simulink model "Formation_FMS2"  (R2022b)
settings: Solver=FixedStepDiscrete  StartTime=0.0  StopTime=10.0  FixedStep=FMS_CONST.dt  RelTol=1e-3
values from neighbouring files (symbols this model uses):
  FMS_PARAM = Simulink.Parameter(FMS_PARAM_VALUE)    [fms_model_init.m]
  FORMATION_PARAM = Simulink.Parameter(FORMATION_PARAM_VALUE)    [fms_model_init.m]
undefined symbols (not defined in the file or in its folder): ax_cmd, ay_cmd, CONTROL_PARAM, DiscIntNeverNeededParam, PilotMode, state, VehicleState, vh_cmd
libraries: FC_Lib x51, simulink x16
(part 2 of 3)

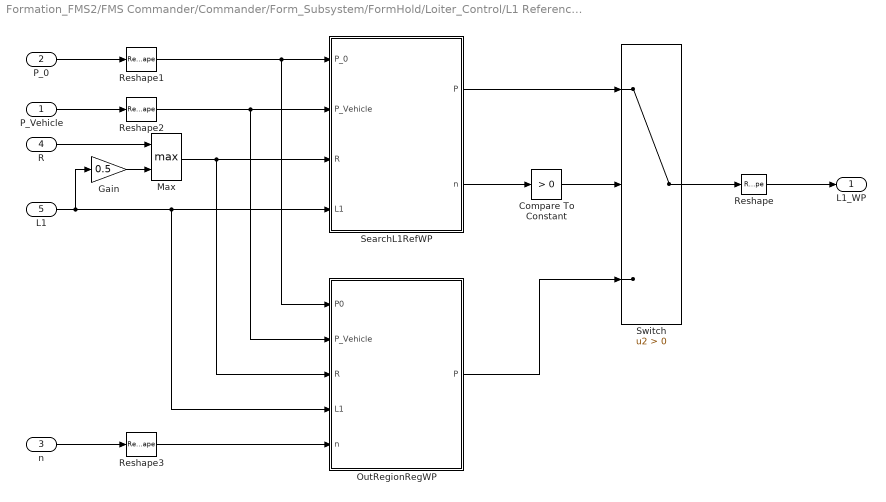
== system Formation_FMS2/FMS Commander/Commander/Form_Subsystem/FormHold/Loiter_Control/L1 Reference WP ==
  P_Vehicle : Inport
  P_0 : Inport  Port=2
  n : Inport  Port=3
  R : Inport  Port=4
  L1 : Inport  Port=5
  Compare To Constant : simulink/Logic and Bit Operations/Compare To Constant  relop=>  const=0  OutDataTypeStr=boolean
  Gain : Gain  Gain=0.5
  Max : MinMax  Function=max  Inputs=2
  OutRegionRegWP : MATLAB Function  TreatAsAtomicUnit=on
  Reshape : Reshape  OutputDimensionality=Customize  OutputDimensions=[2,1]
  Reshape1 : Reshape  OutputDimensionality=Column vector (2-D)
  Reshape2 : Reshape  OutputDimensionality=Column vector (2-D)
  Reshape3 : Reshape  OutputDimensionality=Column vector (2-D)
  SearchL1RefWP : MATLAB Function  TreatAsAtomicUnit=on
  Switch : Switch  Criteria=u2 > Threshold  SaturateOnIntegerOverflow=off  InputSameDT=off
  L1_WP : Outport  VectorParamsAs1DForOutWhenUnconnected=off
  wires:
  Reshape/1 -> L1_WP/1
  Compare To Constant/1 -> Switch/2
  SearchL1RefWP/2(n) -> Compare To Constant/1
  OutRegionRegWP/1(P) -> Switch/3
  Switch/1 -> Reshape/1
  SearchL1RefWP/1(P) -> Switch/1
  P_0/1 -> Reshape1/1
  P_Vehicle/1 -> Reshape2/1
  Max/1 -> OutRegionRegWP/3(R), SearchL1RefWP/3(R)
  L1/1 -> Gain/1, OutRegionRegWP/4(L1), SearchL1RefWP/4(L1)
  Reshape1/1 -> OutRegionRegWP/1(P0), SearchL1RefWP/1(P_0)
  Reshape2/1 -> OutRegionRegWP/2(P_Vehicle), SearchL1RefWP/2(P_Vehicle)
  n/1 -> Reshape3/1
  Reshape3/1 -> OutRegionRegWP/5(n)
  R/1 -> Max/1
  Gain/1 -> Max/2

== system Formation_FMS2/FMS Commander/Commander/Form_Subsystem/FormHold/Loiter_Control/L1_Core ==
  p_vehicle : Inport
  L1_WP : Inport  Port=2
  L1 : Inport  Port=3
  Vg : Inport  Port=4
  L1_Lateral_Acceleration : Subsystem
  Subtract : Sum  Inputs=+-
  ay_cmd_mPs2 : Outport  VectorParamsAs1DForOutWhenUnconnected=off
  wires:
  L1_WP/1 -> Subtract/1
  p_vehicle/1 -> Subtract/2
  L1/1 -> L1_Lateral_Acceleration/1(L1)
  Vg/1 -> L1_Lateral_Acceleration/2(Vg)
  Subtract/1 -> L1_Lateral_Acceleration/3(l1_path)
  L1_Lateral_Acceleration/1(l1_a_cmd) -> ay_cmd_mPs2/1

== system Formation_FMS2/FMS Commander/Commander/Form_Subsystem/FormHold/Loiter_Control/Reference_Point ==
  FMS_In : Inport
  Bus Selector1 : BusSelector  OutputSignals=Cmd_In.cur_waypoint
  Bus Selector2 : BusSelector  OutputSignals=INS_Out.vn,INS_Out.ve
  Bus Selector3 : BusSelector  OutputSignals=INS_Out.x_R,INS_Out.y_R
  Mux1 : Mux  Inputs=2
  Mux2 : Mux  Inputs=2
  Selector : Selector  InputPortWidth=3  IndexOptions=Index vector (dialog)  Indices=[1 2]  OutputSizes=1
  Vector Normalize : FC_Lib/Math/Vector Normalize
      settings: SourceProductName=Flight Control Toolbox
  start_vel : Delay  DelayLength=1  InitialConditionSource=Input port
      settings: InputPortMap=u0,p4
  p_vehicle : Outport  VectorParamsAs1DForOutWhenUnconnected=off
  p_0 : Outport  Port=2  VectorParamsAs1DForOutWhenUnconnected=off
  n : Outport  Port=3  VectorParamsAs1DForOutWhenUnconnected=off
  wires:
  Bus Selector2/2 -> Mux1/2  "<ve>"
  start_vel/1 -> Vector Normalize/1, start_vel/1
  Bus Selector2/1 -> Mux1/1  "<vn>"
  Vector Normalize/1 -> n/1
  FMS_In/1 -> Bus Selector3/1, Bus Selector2/1, Bus Selector1/1
  Mux1/1 -> start_vel/2
  Bus Selector3/1 -> Mux2/1  "<x_R>"
  Bus Selector3/2 -> Mux2/2  "<y_R>"
  Mux2/1 -> p_vehicle/1
  Bus Selector1/1 -> Selector/1  "<cur_waypoint>"
  Selector/1 -> p_0/1

== system Formation_FMS2/FMS Commander/Commander/Form_Subsystem/FormMission/FormMission_SubSystem/Formation_Controller ==
  note: TODO
  FMS_In : Inport
  Bus Selector : BusSelector  OutputSignals=Cmd_In.form_valid
  Bus Selector1 : BusSelector  OutputSignals=Formation_Cross.x_R,Formation_Cross.y_R,Formation_Cross.h_R,Formation_Cross.vn,Formation_Cross.ve,Formation_Cross.vd
  Bus Selector2 : BusSelector  OutputSignals=INS_Out.vn,INS_Out.ve
  Bus Selector3 : BusSelector  OutputSignals=INS_Out.psi
  Consensus Controller : FC_Lib/Fromation/Consensus Controller  uav_id=uav_id  adj_matrix=FORMATION_PARAM.ADJ_MARTIX  rel_x=FORMATION_PARAM.REL_X_MATRIX  rel_y=FORMATION_PARAM.REL_Y_MATRIX  rel_z=FORMATION_PARAM.REL_Z_MATRIX  damp=FORMATION_PARAM.LATERAL_DAMP  period=FORMATION_PARAM.LATERAL_PERIOD  vtrim=CONTROL_PARAM.FW_AIRSPD_TRIM  vmax=CONTROL_PARAM.FW_AIRSPD_MAX  vmin=CONTROL_PARAM.FW_AIRSPD_MIN  pos_kp=FORMATION_PARAM.FORM_POS_KP  vel_kp=FORMATION_PARAM.FORM_VEL_KP  pos_kd=FORMATION_PARAM.FORM_POS_KD
      settings: LibrarySourceBlock=|
      | simulink/User-Defined
      | Functions/MATLAB Function
  Mux : Mux  Inputs=2
  Saturation : Saturate  UpperLimit=inf  LowerLimit=-inf
  Saturation1 : Saturate  UpperLimit=inf  LowerLimit=-inf
  Saturation2 : Saturate  UpperLimit=inf  LowerLimit=-inf
  Vector Concatenate : Concatenate  NumInputs=3  Mode=Multidimensional array  ConcatenateDimension=2
  Vector Concatenate1 : Concatenate  NumInputs=3  Mode=Multidimensional array  ConcatenateDimension=2
  ux_cmd : Outport
  uy_cmd : Outport  Port=2
  uz_cmd : Outport  Port=3
  wires:
  Bus Selector1/2 -> Vector Concatenate/2  "<y_R>"
  Bus Selector/1 -> Consensus Controller/1  "<form_valid>"
  Bus Selector1/4 -> Vector Concatenate1/1  "<vn>"
  Consensus Controller/3 -> Saturation2/1
  Bus Selector1/3 -> Vector Concatenate/3  "<h_R>"
  Vector Concatenate/1 -> Consensus Controller/2  "xyz_O_nx3"
  Bus Selector1/5 -> Vector Concatenate1/2  "<ve>"
  Bus Selector1/1 -> Vector Concatenate/1  "<x_R>"
  Vector Concatenate1/1 -> Consensus Controller/3  "vNED_O_nx3"
  Consensus Controller/2 -> Saturation1/1
  Bus Selector1/6 -> Vector Concatenate1/3  "<vd>"
  FMS_In/1 -> Bus Selector/1, Bus Selector1/1, Bus Selector3/1, Bus Selector2/1
  Consensus Controller/1 -> Saturation/1
  Saturation/1 -> ux_cmd/1
  Saturation1/1 -> uy_cmd/1
  Saturation2/1 -> uz_cmd/1
  Bus Selector2/1 -> Mux/1  "<vn>"
  Bus Selector2/2 -> Mux/2  "<ve>"
  Mux/1 -> Consensus Controller/4
  Bus Selector3/1 -> Consensus Controller/5  "<psi>"

== system Formation_FMS2/FMS Commander/Commander/Form_Subsystem/FormMission/FormMission_SubSystem/Leader_Controller ==
  FMS_In : Inport
  Airspeed Hold : Subsystem
  Altitude_Hold : Subsystem
  FormRadiusLimit : Subsystem
  Position Command : Subsystem
  ax_cmd : Outport
  ay_cmd : Outport  Port=2
  vh_cmd : Outport  Port=3
  wires:
  FMS_In/1 -> Airspeed Hold/1(FMS_In), Altitude_Hold/1(FMS_In), Position Command/1(FMS_In)
  Altitude_Hold/1(vh_cmd) -> vh_cmd/1
  Airspeed Hold/1(ax_cmd) -> ax_cmd/1
  Position Command/1(ay_cmd) -> FormRadiusLimit/1(u)
  FormRadiusLimit/1(y) -> ay_cmd/1

== system Formation_FMS2/FMS Commander/Commander/Hold/Loiter_Control/L1_Core/L1_Lateral_Acceleration ==
  L1 : Inport
  Vg : Inport  Port=2
  l1_path : Inport  Port=3
  Divide : Product  Inputs=*/
  Gain : Gain  Gain=2
  Included Angle : Subsystem
  Multiply1 : Product
  Saturation : Saturate  UpperLimit=pi/2  LowerLimit=-pi/2
  Sin : Trigonometry
  Square : Math  Operator=square  SignedPower=on
  Vector Modulus : FC_Lib/Math/Vector Modulus
      settings: SourceProductName=Flight Control Toolbox
  Vector Normalize : FC_Lib/Math/Vector Normalize
      settings: SourceProductName=Flight Control Toolbox
  Vector Normalize1 : FC_Lib/Math/Vector Normalize
      settings: SourceProductName=Flight Control Toolbox
  l1_a_cmd : Outport  VectorParamsAs1DForOutWhenUnconnected=off
  wires:
  Vector Normalize/1 -> Included Angle/1(vec1)
  Included Angle/1(angle_rad) -> Saturation/1  "L1_alpha"
  Multiply1/1 -> Divide/1
  Divide/1 -> l1_a_cmd/1  "l1_a_cmd"
  Vector Normalize1/1 -> Included Angle/2(vec2)
  Sin/1 -> Multiply1/1  "sin_alpha"
  l1_path/1 -> Vector Normalize1/1
  Saturation/1 -> Sin/1
  Vg/1 -> Vector Normalize/1, Vector Modulus/1
  Square/1 -> Gain/1
  Gain/1 -> Multiply1/2
  L1/1 -> Divide/2
  Vector Modulus/1 -> Square/1

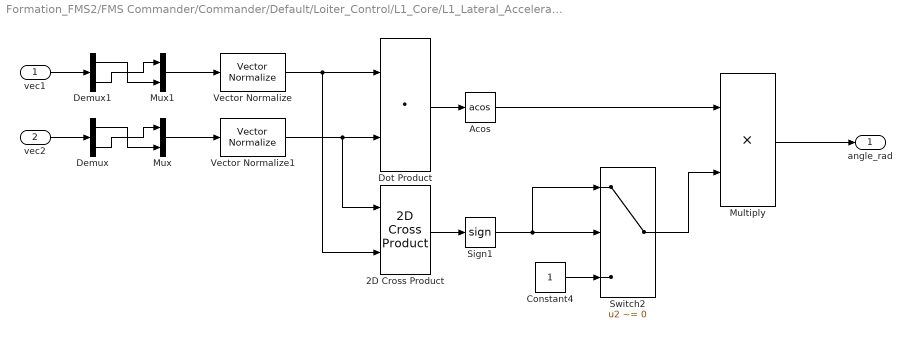
== system Formation_FMS2/FMS Commander/Commander/Default/Loiter_Control/L1_Core/L1_Lateral_Acceleration/Included Angle ==
  vec1 : Inport
  vec2 : Inport  Port=2
  2D Cross Product : FC_Lib/Math/2D Cross Product
      settings: SourceProductName=Flight Control Toolbox
  Acos : Trigonometry  Operator=acos
  Constant4 : Constant  OutDataTypeStr=single
  Demux : Demux  Outputs=2
  Demux1 : Demux  Outputs=2
  Dot Product : DotProduct  OutDataTypeStr=Inherit: Inherit via internal rule
  Multiply : Product
  Mux : Mux  Inputs=2
  Mux1 : Mux  Inputs=2
  Sign1 : Signum
  Switch2 : Switch  Criteria=u2 ~= 0  SaturateOnIntegerOverflow=off  InputSameDT=off
  Vector Normalize : FC_Lib/Math/Vector Normalize
      settings: SourceProductName=Flight Control Toolbox
  Vector Normalize1 : FC_Lib/Math/Vector Normalize
      settings: SourceProductName=Flight Control Toolbox
  angle_rad : Outport  VectorParamsAs1DForOutWhenUnconnected=off
  wires:
  Dot Product/1 -> Acos/1
  Demux1/1 -> Mux1/2
  Mux1/1 -> Vector Normalize/1
  Demux1/2 -> Mux1/1
  Sign1/1 -> Switch2/1, Switch2/2
  Vector Normalize1/1 -> Dot Product/2, 2D Cross Product/1
  Demux/2 -> Mux/1
  Vector Normalize/1 -> Dot Product/1, 2D Cross Product/2
  2D Cross Product/1 -> Sign1/1
  Multiply/1 -> angle_rad/1
  vec1/1 -> Demux1/1
  Demux/1 -> Mux/2
  Constant4/1 -> Switch2/3
  vec2/1 -> Demux/1
  Mux/1 -> Vector Normalize1/1
  Acos/1 -> Multiply/1
  Switch2/1 -> Multiply/2

== system Formation_FMS2/FMS Commander/Commander/Form_Subsystem/Default/Loiter_Control/L1_Core/L1_Lateral_Acceleration ==
  L1 : Inport
  Vg : Inport  Port=2
  l1_path : Inport  Port=3
  Divide : Product  Inputs=*/
  Gain : Gain  Gain=2
  Included Angle : Subsystem
  Multiply1 : Product
  Saturation : Saturate  UpperLimit=pi/2  LowerLimit=-pi/2
  Sin : Trigonometry
  Square : Math  Operator=square  SignedPower=on
  Vector Modulus : FC_Lib/Math/Vector Modulus
      settings: SourceProductName=Flight Control Toolbox
  Vector Normalize : FC_Lib/Math/Vector Normalize
      settings: SourceProductName=Flight Control Toolbox
  Vector Normalize1 : FC_Lib/Math/Vector Normalize
      settings: SourceProductName=Flight Control Toolbox
  l1_a_cmd : Outport  VectorParamsAs1DForOutWhenUnconnected=off
  wires:
  Vector Modulus/1 -> Square/1
  L1/1 -> Divide/2
  Gain/1 -> Multiply1/2
  Square/1 -> Gain/1
  Vg/1 -> Vector Modulus/1, Vector Normalize/1
  Saturation/1 -> Sin/1
  l1_path/1 -> Vector Normalize1/1
  Sin/1 -> Multiply1/1  "sin_alpha"
  Vector Normalize1/1 -> Included Angle/2(vec2)
  Divide/1 -> l1_a_cmd/1  "l1_a_cmd"
  Multiply1/1 -> Divide/1
  Included Angle/1(angle_rad) -> Saturation/1  "L1_alpha"
  Vector Normalize/1 -> Included Angle/1(vec1)

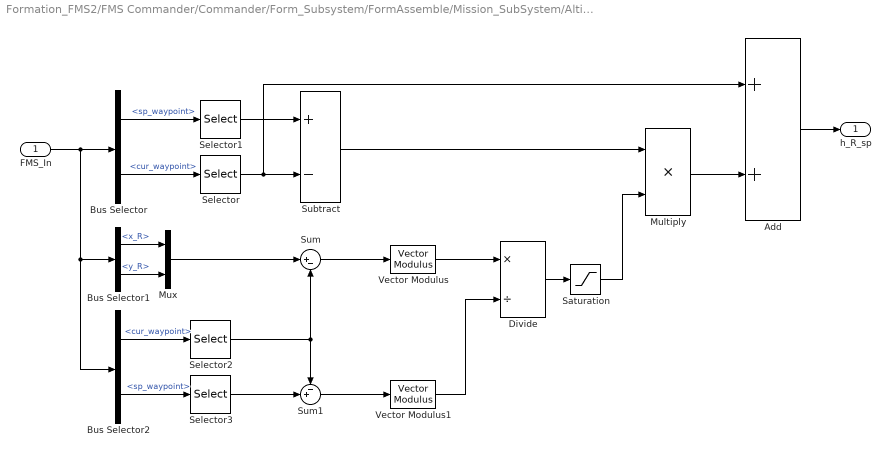
== system Formation_FMS2/FMS Commander/Commander/Form_Subsystem/FormAssemble/Mission_SubSystem/Altitude Control/Target Height ==
  FMS_In : Inport
  Add : Sum
  Bus Selector : BusSelector  OutputSignals=Cmd_In.sp_waypoint,Cmd_In.cur_waypoint
  Bus Selector1 : BusSelector  OutputSignals=INS_Out.x_R,INS_Out.y_R
  Bus Selector2 : BusSelector  OutputSignals=Cmd_In.cur_waypoint,Cmd_In.sp_waypoint
  Divide : Product  Inputs=*/
  Multiply : Product
  Mux : Mux  Inputs=2
  Saturation : Saturate  UpperLimit=1  LowerLimit=0
  Selector : Selector  InputPortWidth=3  IndexOptions=Index vector (dialog)  Indices=3  OutputSizes=1
  Selector1 : Selector  InputPortWidth=3  IndexOptions=Index vector (dialog)  Indices=3  OutputSizes=1
  Selector2 : Selector  InputPortWidth=3  IndexOptions=Index vector (dialog)  Indices=[1 2]  OutputSizes=1
  Selector3 : Selector  InputPortWidth=3  IndexOptions=Index vector (dialog)  Indices=[1 2]  OutputSizes=1
  Subtract : Sum  Inputs=+-
  Sum : Sum  Inputs=|+-
  Sum1 : Sum  Inputs=-+|
  Vector Modulus : FC_Lib/Math/Vector Modulus
      settings: SourceProductName=Flight Control Toolbox
  Vector Modulus1 : FC_Lib/Math/Vector Modulus
      settings: SourceProductName=Flight Control Toolbox
  h_R_sp : Outport  VectorParamsAs1DForOutWhenUnconnected=off
  wires:
  Multiply/1 -> Add/2
  Bus Selector1/1 -> Mux/1  "<x_R>"
  Bus Selector/1 -> Selector1/1  "<sp_waypoint>"
  Vector Modulus1/1 -> Divide/2
  Sum1/1 -> Vector Modulus1/1
  Sum/1 -> Vector Modulus/1
  Selector2/1 -> Sum1/1, Sum/2
  FMS_In/1 -> Bus Selector2/1, Bus Selector1/1, Bus Selector/1
  Bus Selector2/2 -> Selector3/1  "<sp_waypoint>"
  Vector Modulus/1 -> Divide/1
  Bus Selector1/2 -> Mux/2  "<y_R>"
  Bus Selector2/1 -> Selector2/1  "<cur_waypoint>"
  Selector1/1 -> Subtract/1
  Mux/1 -> Sum/1
  Subtract/1 -> Multiply/1
  Divide/1 -> Saturation/1
  Selector3/1 -> Sum1/2
  Bus Selector/2 -> Selector/1  "<cur_waypoint>"
  Selector/1 -> Add/1, Subtract/2
  Saturation/1 -> Multiply/2
  Add/1 -> h_R_sp/1

== system Formation_FMS2/FMS Commander/Commander/Form_Subsystem/FormAssemble/Mission_SubSystem/Position Command/L1 Control ==
  p1 : Inport
  p2 : Inport  Port=2
  p3 : Inport  Port=3
  FMS_In : Inport  Port=4
  Bus Selector1 : BusSelector  OutputSignals=INS_Out.vn,INS_Out.ve
  L1 : Constant  Value=FMS_PARAM.L1  OutDataTypeStr=single
  L1 Reference WP : Subsystem
  L1_Core : Subsystem
  Mux : Mux  Inputs=2
  Saturation1 : Saturate  UpperLimit=FMS_PARAM.ACC_Y_LIM  LowerLimit=-FMS_PARAM.ACC_Y_LIM
  ay_cmd_mPs2 : Outport  VectorParamsAs1DForOutWhenUnconnected=off
  wires:
  p3/1 -> L1_Core/1(p_vehicle), L1 Reference WP/3(P3)
  p2/1 -> L1 Reference WP/2(P2)
  p1/1 -> L1 Reference WP/1(P1)
  L1/1 -> L1_Core/3(L1), L1 Reference WP/4(L1)
  L1 Reference WP/1(L1_WP) -> L1_Core/2(L1_WP)  "L1_WP"
  Mux/1 -> L1_Core/4(Vg)
  Bus Selector1/1 -> Mux/1  "<vn>"
  Bus Selector1/2 -> Mux/2  "<ve>"
  FMS_In/1 -> Bus Selector1/1
  L1_Core/1(ay_cmd_mPs2) -> Saturation1/1
  Saturation1/1 -> ay_cmd_mPs2/1

== system Formation_FMS2/FMS Commander/Commander/Form_Subsystem/FormAssemble/Mission_SubSystem/Position Command/WayPoints ==
  note: P1: path start point
      | P2: path end point
      | P3: vehicle point
  FMS_In : Inport
  Bus Selector : BusSelector  OutputSignals=INS_Out.x_R,INS_Out.y_R
  Bus Selector1 : BusSelector  OutputSignals=Cmd_In.sp_waypoint
  Bus Selector2 : BusSelector  OutputSignals=Cmd_In.cur_waypoint
  Mux : Mux  Inputs=2
  Reshape : Reshape  OutputDimensionality=Customize  OutputDimensions=[2,1]
  Reshape1 : Reshape  OutputDimensionality=Customize  OutputDimensions=[2,1]
  Reshape2 : Reshape  OutputDimensionality=Customize  OutputDimensions=[2,1]
  Selector : Selector  InputPortWidth=3  IndexOptions=Index vector (dialog)  Indices=[1 2]  OutputSizes=1
  Selector1 : Selector  InputPortWidth=3  IndexOptions=Index vector (dialog)  Indices=[1 2]  OutputSizes=1
  p1 : Outport  VectorParamsAs1DForOutWhenUnconnected=off
  p2 : Outport  Port=2  VectorParamsAs1DForOutWhenUnconnected=off
  p3 : Outport  Port=3  VectorParamsAs1DForOutWhenUnconnected=off
  wires:
  Reshape2/1 -> p3/1
  Reshape1/1 -> p1/1
  Reshape/1 -> p2/1
  Bus Selector/2 -> Mux/2  "<y_R>"
  Bus Selector/1 -> Mux/1  "<x_R>"
  Mux/1 -> Reshape2/1
  FMS_In/1 -> Bus Selector2/1, Bus Selector1/1, Bus Selector/1
  Bus Selector1/1 -> Selector/1  "<sp_waypoint>"
  Selector/1 -> Reshape/1
  Bus Selector2/1 -> Selector1/1  "<cur_waypoint>"
  Selector1/1 -> Reshape1/1

== system Formation_FMS2/FMS Commander/Commander/Form_Subsystem/FormDisband/Loiter_Control/L1_Core/L1_Lateral_Acceleration ==
  L1 : Inport
  Vg : Inport  Port=2
  l1_path : Inport  Port=3
  Divide : Product  Inputs=*/
  Gain : Gain  Gain=2
  Included Angle : Subsystem
  Multiply1 : Product
  Saturation : Saturate  UpperLimit=pi/2  LowerLimit=-pi/2
  Sin : Trigonometry
  Square : Math  Operator=square  SignedPower=on
  Vector Modulus : FC_Lib/Math/Vector Modulus
      settings: SourceProductName=Flight Control Toolbox
  Vector Normalize : FC_Lib/Math/Vector Normalize
      settings: SourceProductName=Flight Control Toolbox
  Vector Normalize1 : FC_Lib/Math/Vector Normalize
      settings: SourceProductName=Flight Control Toolbox
  l1_a_cmd : Outport  VectorParamsAs1DForOutWhenUnconnected=off
  wires:
  Vector Modulus/1 -> Square/1
  L1/1 -> Divide/2
  Gain/1 -> Multiply1/2
  Square/1 -> Gain/1
  Vg/1 -> Vector Modulus/1, Vector Normalize/1
  Saturation/1 -> Sin/1
  l1_path/1 -> Vector Normalize1/1
  Sin/1 -> Multiply1/1  "sin_alpha"
  Vector Normalize1/1 -> Included Angle/2(vec2)
  Divide/1 -> l1_a_cmd/1  "l1_a_cmd"
  Multiply1/1 -> Divide/1
  Included Angle/1(angle_rad) -> Saturation/1  "L1_alpha"
  Vector Normalize/1 -> Included Angle/1(vec1)

== system Formation_FMS2/FMS Commander/Commander/Form_Subsystem/FormHold/Loiter_Control/L1_Core/L1_Lateral_Acceleration ==
  L1 : Inport
  Vg : Inport  Port=2
  l1_path : Inport  Port=3
  Divide : Product  Inputs=*/
  Gain : Gain  Gain=2
  Included Angle : Subsystem
  Multiply1 : Product
  Saturation : Saturate  UpperLimit=pi/2  LowerLimit=-pi/2
  Sin : Trigonometry
  Square : Math  Operator=square  SignedPower=on
  Vector Modulus : FC_Lib/Math/Vector Modulus
      settings: SourceProductName=Flight Control Toolbox
  Vector Normalize : FC_Lib/Math/Vector Normalize
      settings: SourceProductName=Flight Control Toolbox
  Vector Normalize1 : FC_Lib/Math/Vector Normalize
      settings: SourceProductName=Flight Control Toolbox
  l1_a_cmd : Outport  VectorParamsAs1DForOutWhenUnconnected=off
  wires:
  Vector Normalize/1 -> Included Angle/1(vec1)
  Included Angle/1(angle_rad) -> Saturation/1  "L1_alpha"
  Multiply1/1 -> Divide/1
  Divide/1 -> l1_a_cmd/1  "l1_a_cmd"
  Vector Normalize1/1 -> Included Angle/2(vec2)
  Sin/1 -> Multiply1/1  "sin_alpha"
  l1_path/1 -> Vector Normalize1/1
  Saturation/1 -> Sin/1
  Vg/1 -> Vector Normalize/1, Vector Modulus/1
  Square/1 -> Gain/1
  Gain/1 -> Multiply1/2
  L1/1 -> Divide/2
  Vector Modulus/1 -> Square/1

== system Formation_FMS2/FMS Commander/Commander/Form_Subsystem/FormMission/FormMission_SubSystem/Leader_Controller/Airspeed Hold ==
  FMS_In : Inport
  Bus Selector : BusSelector  OutputSignals=INS_Out.airspeed
  Constant : Constant  Value=FMS_PARAM.FW_AIRSPD_TRIM
  Gain : Gain  Gain=FMS_PARAM.AIRSPD_P
  Sum : Sum  Inputs=-+|
  ax_cmd : Outport
  wires:
  Sum/1 -> Gain/1  "v_error"
  Gain/1 -> ax_cmd/1  "ax_cmd"
  Constant/1 -> Sum/2
  FMS_In/1 -> Bus Selector/1
  Bus Selector/1 -> Sum/1  "<airspeed>"

== system Formation_FMS2/FMS Commander/Commander/Form_Subsystem/FormMission/FormMission_SubSystem/Leader_Controller/Altitude_Hold ==
  FMS_In : Inport
  Bus Selector2 : BusSelector  OutputSignals=INS_Out.h_R
  Constant : Constant  Value=FMS_PARAM.FW_HEIGHT_TRIM
  Delay : Delay  DelayLength=1  InitialConditionSource=Input port
      settings: InputPortMap=u0,p4
  Gain2 : Gain  Gain=FMS_PARAM.Z_P  OutDataTypeStr=single
  Saturation : Saturate  UpperLimit=CONTROL_PARAM.FW_T_CLMB_MAX  LowerLimit=-CONTROL_PARAM.FW_T_SINK_MAX
  Sum : Sum  Inputs=-+|
  vh_cmd : Outport  VectorParamsAs1DForOutWhenUnconnected=off
  wires:
  Gain2/1 -> Saturation/1
  Bus Selector2/1 -> Sum/1  "<h_R>"
  Sum/1 -> Gain2/1  "h_err_R"
  Delay/1 -> Sum/2, Delay/1  "h_cmd_R"
  FMS_In/1 -> Bus Selector2/1
  Saturation/1 -> vh_cmd/1
  Constant/1 -> Delay/2

== system Formation_FMS2/FMS Commander/Commander/Form_Subsystem/FormMission/FormMission_SubSystem/Leader_Controller/FormRadiusLimit ==
  note: R_{leader} > \frac{D_{lateral} \times V_{leader}}{min(V_{max} - V_{leader}, V_{leader} - V_{min})}
  u : Inport
  Divide : Product  Inputs=*/
  Gain : Gain  Gain=-1
  Satefy : Gain  Gain=FMS_PARAM.FW_RADIUS_RATIO
  Saturation Dynamic : simulink/Discontinuities/Saturation Dynamic  OutMin=[]  OutMax=[]  OutDataTypeStr=Inherit: Same as second input  OutDataType=fixdt(1, 16)  OutScaling=2^-10  DoSatur=off
  min_radius : MATLAB Function  TreatAsAtomicUnit=on  mask{dis_lat=FORMATION_PARAM.REL_Y_MATRIX, vtrim=CONTROL_PARAM.FW_AIRSPD_TRIM, vmax=CONTROL_PARAM.FW_AIRSPD_MAX, vmin=CONTROL_PARAM.FW_AIRSPD_MIN}
  v^2 : Constant  Value=CONTROL_PARAM.FW_AIRSPD_TRIM*CONTROL_PARAM.FW_AIRSPD_TRIM
  y : Outport
  wires:
  v^2/1 -> Divide/1
  Divide/1 -> Saturation Dynamic/1, Gain/1
  u/1 -> Saturation Dynamic/2
  Gain/1 -> Saturation Dynamic/3
  Saturation Dynamic/1 -> y/1
  Satefy/1 -> Divide/2
  min_radius/1(y) -> Satefy/1

== system Formation_FMS2/FMS Commander/Commander/Form_Subsystem/FormMission/FormMission_SubSystem/Leader_Controller/Position Command ==
  FMS_In : Inport
  L1 Control : Subsystem
  WayPoints : Subsystem
  ay_cmd : Outport  VectorParamsAs1DForOutWhenUnconnected=off
  wires:
  FMS_In/1 -> L1 Control/4(FMS_In), WayPoints/1(FMS_In)
  WayPoints/2(p2) -> L1 Control/2(p2)
  WayPoints/3(p3) -> L1 Control/3(p3)
  WayPoints/1(p1) -> L1 Control/1(p1)
  L1 Control/1(ay_cmd_mPs2) -> ay_cmd/1

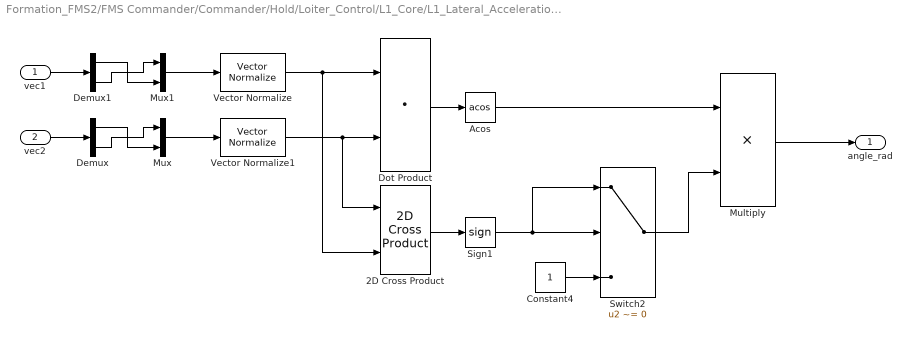
== system Formation_FMS2/FMS Commander/Commander/Hold/Loiter_Control/L1_Core/L1_Lateral_Acceleration/Included Angle ==
  vec1 : Inport
  vec2 : Inport  Port=2
  2D Cross Product : FC_Lib/Math/2D Cross Product
      settings: SourceProductName=Flight Control Toolbox
  Acos : Trigonometry  Operator=acos
  Constant4 : Constant  OutDataTypeStr=single
  Demux : Demux  Outputs=2
  Demux1 : Demux  Outputs=2
  Dot Product : DotProduct  OutDataTypeStr=Inherit: Inherit via internal rule
  Multiply : Product
  Mux : Mux  Inputs=2
  Mux1 : Mux  Inputs=2
  Sign1 : Signum
  Switch2 : Switch  Criteria=u2 ~= 0  SaturateOnIntegerOverflow=off  InputSameDT=off
  Vector Normalize : FC_Lib/Math/Vector Normalize
      settings: SourceProductName=Flight Control Toolbox
  Vector Normalize1 : FC_Lib/Math/Vector Normalize
      settings: SourceProductName=Flight Control Toolbox
  angle_rad : Outport  VectorParamsAs1DForOutWhenUnconnected=off
  wires:
  Switch2/1 -> Multiply/2
  Acos/1 -> Multiply/1
  Mux/1 -> Vector Normalize1/1
  vec2/1 -> Demux/1
  Constant4/1 -> Switch2/3
  Demux/1 -> Mux/2
  vec1/1 -> Demux1/1
  Multiply/1 -> angle_rad/1
  2D Cross Product/1 -> Sign1/1
  Vector Normalize/1 -> 2D Cross Product/2, Dot Product/1
  Demux/2 -> Mux/1
  Vector Normalize1/1 -> 2D Cross Product/1, Dot Product/2
  Sign1/1 -> Switch2/2, Switch2/1
  Demux1/2 -> Mux1/1
  Mux1/1 -> Vector Normalize/1
  Demux1/1 -> Mux1/2
  Dot Product/1 -> Acos/1

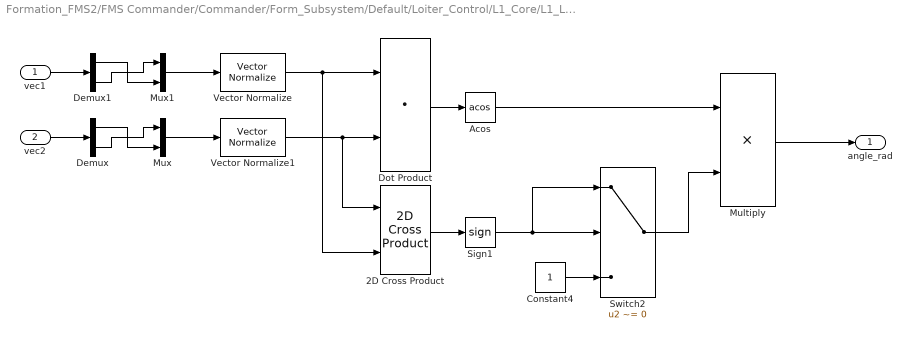
== system Formation_FMS2/FMS Commander/Commander/Form_Subsystem/Default/Loiter_Control/L1_Core/L1_Lateral_Acceleration/Included Angle ==
  vec1 : Inport
  vec2 : Inport  Port=2
  2D Cross Product : FC_Lib/Math/2D Cross Product
      settings: SourceProductName=Flight Control Toolbox
  Acos : Trigonometry  Operator=acos
  Constant4 : Constant  OutDataTypeStr=single
  Demux : Demux  Outputs=2
  Demux1 : Demux  Outputs=2
  Dot Product : DotProduct  OutDataTypeStr=Inherit: Inherit via internal rule
  Multiply : Product
  Mux : Mux  Inputs=2
  Mux1 : Mux  Inputs=2
  Sign1 : Signum
  Switch2 : Switch  Criteria=u2 ~= 0  SaturateOnIntegerOverflow=off  InputSameDT=off
  Vector Normalize : FC_Lib/Math/Vector Normalize
      settings: SourceProductName=Flight Control Toolbox
  Vector Normalize1 : FC_Lib/Math/Vector Normalize
      settings: SourceProductName=Flight Control Toolbox
  angle_rad : Outport  VectorParamsAs1DForOutWhenUnconnected=off
  wires:
  Dot Product/1 -> Acos/1
  Demux1/1 -> Mux1/2
  Mux1/1 -> Vector Normalize/1
  Demux1/2 -> Mux1/1
  Sign1/1 -> Switch2/1, Switch2/2
  Vector Normalize1/1 -> Dot Product/2, 2D Cross Product/1
  Demux/2 -> Mux/1
  Vector Normalize/1 -> Dot Product/1, 2D Cross Product/2
  2D Cross Product/1 -> Sign1/1
  Multiply/1 -> angle_rad/1
  vec1/1 -> Demux1/1
  Demux/1 -> Mux/2
  Constant4/1 -> Switch2/3
  vec2/1 -> Demux/1
  Mux/1 -> Vector Normalize1/1
  Acos/1 -> Multiply/1
  Switch2/1 -> Multiply/2

== system Formation_FMS2/FMS Commander/Commander/Form_Subsystem/FormAssemble/Mission_SubSystem/Position Command/L1 Control/L1 Reference WP ==
  P1 : Inport
  P2 : Inport  Port=2
  P3 : Inport  Port=3
  L1 : Inport  Port=4
  Compare To Constant : simulink/Logic and Bit Operations/Compare To Constant  relop=>=  const=0  OutDataTypeStr=boolean
  Compare To Constant1 : simulink/Logic and Bit Operations/Compare To Constant  relop=>  const=0  OutDataTypeStr=boolean
  NearbyRefWP : MATLAB Function  TreatAsAtomicUnit=on
  OutRegionRegWP : MATLAB Function  TreatAsAtomicUnit=on
  Reshape : Reshape  OutputDimensionality=Customize  OutputDimensions=[2,1]
  SearchL1RefWP : MATLAB Function  TreatAsAtomicUnit=on
  Switch : Switch  Criteria=u2 > Threshold  SaturateOnIntegerOverflow=off  InputSameDT=off
  Switch1 : Switch  Criteria=u2 > Threshold  SaturateOnIntegerOverflow=off  InputSameDT=off
  L1_WP : Outport  VectorParamsAs1DForOutWhenUnconnected=off
  wires:
  Reshape/1 -> L1_WP/1
  Compare To Constant/1 -> Switch/2
  NearbyRefWP/2(d) -> Compare To Constant1/1  "distance"
  SearchL1RefWP/2(u) -> Compare To Constant/1  "l1_u"
  Compare To Constant1/1 -> Switch1/2
  P1/1 -> SearchL1RefWP/1(P1), OutRegionRegWP/1(P1)
  P2/1 -> SearchL1RefWP/2(P2), NearbyRefWP/1(P2), OutRegionRegWP/2(P2)
  P3/1 -> NearbyRefWP/2(P3), SearchL1RefWP/3(P3), OutRegionRegWP/3(P3)
  Switch/1 -> Switch1/3
  L1/1 -> SearchL1RefWP/4(L1), NearbyRefWP/3(L1)
  OutRegionRegWP/1(P) -> Switch/3  "out_WP"
  Switch1/1 -> Reshape/1
  SearchL1RefWP/1(P) -> Switch/1  "L1_Ref_P"
  NearbyRefWP/1(P) -> Switch1/1  "NearbyWP"

== system Formation_FMS2/FMS Commander/Commander/Form_Subsystem/FormAssemble/Mission_SubSystem/Position Command/L1 Control/L1_Core ==
  p_vehicle : Inport
  L1_WP : Inport  Port=2
  L1 : Inport  Port=3
  Vg : Inport  Port=4
  L1_Lateral_Acceleration : Subsystem
  Subtract : Sum  Inputs=+-
  ay_cmd_mPs2 : Outport  VectorParamsAs1DForOutWhenUnconnected=off
  wires:
  L1_WP/1 -> Subtract/1
  p_vehicle/1 -> Subtract/2
  L1/1 -> L1_Lateral_Acceleration/1(L1)
  Vg/1 -> L1_Lateral_Acceleration/2(Vg)
  Subtract/1 -> L1_Lateral_Acceleration/3(l1_path)
  L1_Lateral_Acceleration/1(l1_a_cmd) -> ay_cmd_mPs2/1

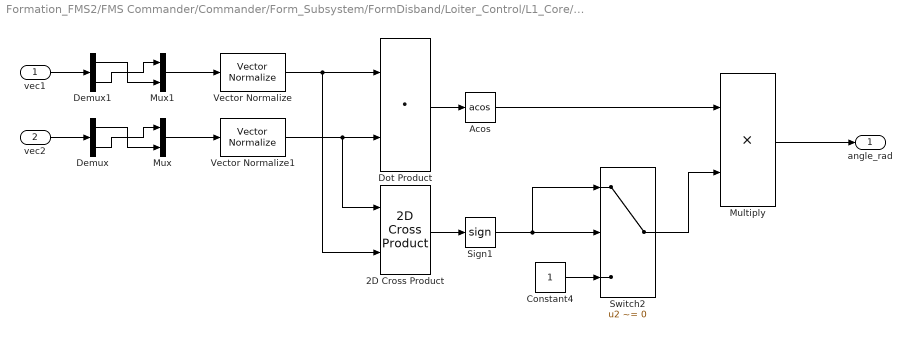
== system Formation_FMS2/FMS Commander/Commander/Form_Subsystem/FormDisband/Loiter_Control/L1_Core/L1_Lateral_Acceleration/Included Angle ==
  vec1 : Inport
  vec2 : Inport  Port=2
  2D Cross Product : FC_Lib/Math/2D Cross Product
      settings: SourceProductName=Flight Control Toolbox
  Acos : Trigonometry  Operator=acos
  Constant4 : Constant  OutDataTypeStr=single
  Demux : Demux  Outputs=2
  Demux1 : Demux  Outputs=2
  Dot Product : DotProduct  OutDataTypeStr=Inherit: Inherit via internal rule
  Multiply : Product
  Mux : Mux  Inputs=2
  Mux1 : Mux  Inputs=2
  Sign1 : Signum
  Switch2 : Switch  Criteria=u2 ~= 0  SaturateOnIntegerOverflow=off  InputSameDT=off
  Vector Normalize : FC_Lib/Math/Vector Normalize
      settings: SourceProductName=Flight Control Toolbox
  Vector Normalize1 : FC_Lib/Math/Vector Normalize
      settings: SourceProductName=Flight Control Toolbox
  angle_rad : Outport  VectorParamsAs1DForOutWhenUnconnected=off
  wires:
  Dot Product/1 -> Acos/1
  Demux1/1 -> Mux1/2
  Mux1/1 -> Vector Normalize/1
  Demux1/2 -> Mux1/1
  Sign1/1 -> Switch2/1, Switch2/2
  Vector Normalize1/1 -> Dot Product/2, 2D Cross Product/1
  Demux/2 -> Mux/1
  Vector Normalize/1 -> Dot Product/1, 2D Cross Product/2
  2D Cross Product/1 -> Sign1/1
  Multiply/1 -> angle_rad/1
  vec1/1 -> Demux1/1
  Demux/1 -> Mux/2
  Constant4/1 -> Switch2/3
  vec2/1 -> Demux/1
  Mux/1 -> Vector Normalize1/1
  Acos/1 -> Multiply/1
  Switch2/1 -> Multiply/2

== system Formation_FMS2/FMS Commander/Commander/Form_Subsystem/FormHold/Loiter_Control/L1_Core/L1_Lateral_Acceleration/Included Angle ==
  vec1 : Inport
  vec2 : Inport  Port=2
  2D Cross Product : FC_Lib/Math/2D Cross Product
      settings: SourceProductName=Flight Control Toolbox
  Acos : Trigonometry  Operator=acos
  Constant4 : Constant  OutDataTypeStr=single
  Demux : Demux  Outputs=2
  Demux1 : Demux  Outputs=2
  Dot Product : DotProduct  OutDataTypeStr=Inherit: Inherit via internal rule
  Multiply : Product
  Mux : Mux  Inputs=2
  Mux1 : Mux  Inputs=2
  Sign1 : Signum
  Switch2 : Switch  Criteria=u2 ~= 0  SaturateOnIntegerOverflow=off  InputSameDT=off
  Vector Normalize : FC_Lib/Math/Vector Normalize
      settings: SourceProductName=Flight Control Toolbox
  Vector Normalize1 : FC_Lib/Math/Vector Normalize
      settings: SourceProductName=Flight Control Toolbox
  angle_rad : Outport  VectorParamsAs1DForOutWhenUnconnected=off
  wires:
  Switch2/1 -> Multiply/2
  Acos/1 -> Multiply/1
  Mux/1 -> Vector Normalize1/1
  vec2/1 -> Demux/1
  Constant4/1 -> Switch2/3
  Demux/1 -> Mux/2
  vec1/1 -> Demux1/1
  Multiply/1 -> angle_rad/1
  2D Cross Product/1 -> Sign1/1
  Vector Normalize/1 -> 2D Cross Product/2, Dot Product/1
  Demux/2 -> Mux/1
  Vector Normalize1/1 -> 2D Cross Product/1, Dot Product/2
  Sign1/1 -> Switch2/2, Switch2/1
  Demux1/2 -> Mux1/1
  Mux1/1 -> Vector Normalize/1
  Demux1/1 -> Mux1/2
  Dot Product/1 -> Acos/1

== system Formation_FMS2/FMS Commander/Commander/Form_Subsystem/FormMission/FormMission_SubSystem/Leader_Controller/Position Command/L1 Control ==
  p1 : Inport
  p2 : Inport  Port=2
  p3 : Inport  Port=3
  FMS_In : Inport  Port=4
  Bus Selector1 : BusSelector  OutputSignals=INS_Out.vn,INS_Out.ve
  L1 : Constant  Value=FMS_PARAM.L1  OutDataTypeStr=single
  L1 Reference WP : Subsystem
  L1_Core : Subsystem
  Mux : Mux  Inputs=2
  Saturation1 : Saturate  UpperLimit=FMS_PARAM.ACC_Y_LIM  LowerLimit=-FMS_PARAM.ACC_Y_LIM
  ay_cmd_mPs2 : Outport  VectorParamsAs1DForOutWhenUnconnected=off
  wires:
  p3/1 -> L1_Core/1(p_vehicle), L1 Reference WP/3(P3)
  p2/1 -> L1 Reference WP/2(P2)
  p1/1 -> L1 Reference WP/1(P1)
  L1/1 -> L1_Core/3(L1), L1 Reference WP/4(L1)
  L1 Reference WP/1(L1_WP) -> L1_Core/2(L1_WP)  "L1_WP"
  Mux/1 -> L1_Core/4(Vg)
  Bus Selector1/1 -> Mux/1  "<vn>"
  Bus Selector1/2 -> Mux/2  "<ve>"
  FMS_In/1 -> Bus Selector1/1
  L1_Core/1(ay_cmd_mPs2) -> Saturation1/1
  Saturation1/1 -> ay_cmd_mPs2/1

== system Formation_FMS2/FMS Commander/Commander/Form_Subsystem/FormMission/FormMission_SubSystem/Leader_Controller/Position Command/WayPoints ==
  note: P1: path start point
      | P2: path end point
      | P3: vehicle point
  FMS_In : Inport
  Bus Selector : BusSelector  OutputSignals=INS_Out.x_R,INS_Out.y_R
  Bus Selector1 : BusSelector  OutputSignals=Cmd_In.sp_waypoint
  Bus Selector2 : BusSelector  OutputSignals=Cmd_In.cur_waypoint
  Mux : Mux  Inputs=2
  Reshape : Reshape  OutputDimensionality=Customize  OutputDimensions=[2,1]
  Reshape1 : Reshape  OutputDimensionality=Customize  OutputDimensions=[2,1]
  Reshape2 : Reshape  OutputDimensionality=Customize  OutputDimensions=[2,1]
  Selector : Selector  InputPortWidth=3  IndexOptions=Index vector (dialog)  Indices=[1 2]  OutputSizes=1
  Selector1 : Selector  InputPortWidth=3  IndexOptions=Index vector (dialog)  Indices=[1 2]  OutputSizes=1
  p1 : Outport  VectorParamsAs1DForOutWhenUnconnected=off
  p2 : Outport  Port=2  VectorParamsAs1DForOutWhenUnconnected=off
  p3 : Outport  Port=3  VectorParamsAs1DForOutWhenUnconnected=off
  wires:
  Reshape2/1 -> p3/1
  Reshape1/1 -> p1/1
  Reshape/1 -> p2/1
  Bus Selector/2 -> Mux/2  "<y_R>"
  Bus Selector/1 -> Mux/1  "<x_R>"
  Mux/1 -> Reshape2/1
  FMS_In/1 -> Bus Selector2/1, Bus Selector1/1, Bus Selector/1
  Bus Selector1/1 -> Selector/1  "<sp_waypoint>"
  Selector/1 -> Reshape/1
  Bus Selector2/1 -> Selector1/1  "<cur_waypoint>"
  Selector1/1 -> Reshape1/1

== system Formation_FMS2/FMS Commander/Commander/Form_Subsystem/FormAssemble/Mission_SubSystem/Position Command/L1 Control/L1_Core/L1_Lateral_Acceleration ==
  L1 : Inport
  Vg : Inport  Port=2
  l1_path : Inport  Port=3
  Divide : Product  Inputs=*/
  Gain : Gain  Gain=2
  Included Angle : Subsystem
  Multiply1 : Product
  Saturation : Saturate  UpperLimit=pi/2  LowerLimit=-pi/2
  Sin : Trigonometry
  Square : Math  Operator=square  SignedPower=on
  Vector Modulus : FC_Lib/Math/Vector Modulus
      settings: SourceProductName=Flight Control Toolbox
  Vector Normalize : FC_Lib/Math/Vector Normalize
      settings: SourceProductName=Flight Control Toolbox
  Vector Normalize1 : FC_Lib/Math/Vector Normalize
      settings: SourceProductName=Flight Control Toolbox
  l1_a_cmd : Outport  VectorParamsAs1DForOutWhenUnconnected=off
  wires:
  Vector Normalize/1 -> Included Angle/1(vec1)
  Included Angle/1(angle_rad) -> Saturation/1  "L1_alpha"
  Multiply1/1 -> Divide/1
  Divide/1 -> l1_a_cmd/1  "l1_a_cmd"
  Vector Normalize1/1 -> Included Angle/2(vec2)
  Sin/1 -> Multiply1/1  "sin_alpha"
  l1_path/1 -> Vector Normalize1/1
  Saturation/1 -> Sin/1
  Vg/1 -> Vector Normalize/1, Vector Modulus/1
  Square/1 -> Gain/1
  Gain/1 -> Multiply1/2
  L1/1 -> Divide/2
  Vector Modulus/1 -> Square/1

== system Formation_FMS2/FMS Commander/Commander/Form_Subsystem/FormMission/FormMission_SubSystem/Leader_Controller/Position Command/L1 Control/L1 Reference WP ==
  P1 : Inport
  P2 : Inport  Port=2
  P3 : Inport  Port=3
  L1 : Inport  Port=4
  Compare To Constant : simulink/Logic and Bit Operations/Compare To Constant  relop=>=  const=0  OutDataTypeStr=boolean
  Compare To Constant1 : simulink/Logic and Bit Operations/Compare To Constant  relop=>  const=0  OutDataTypeStr=boolean
  NearbyRefWP : MATLAB Function  TreatAsAtomicUnit=on
  OutRegionRegWP : MATLAB Function  TreatAsAtomicUnit=on
  Reshape : Reshape  OutputDimensionality=Customize  OutputDimensions=[2,1]
  SearchL1RefWP : MATLAB Function  TreatAsAtomicUnit=on
  Switch : Switch  Criteria=u2 > Threshold  SaturateOnIntegerOverflow=off  InputSameDT=off
  Switch1 : Switch  Criteria=u2 > Threshold  SaturateOnIntegerOverflow=off  InputSameDT=off
  L1_WP : Outport  VectorParamsAs1DForOutWhenUnconnected=off
  wires:
  Reshape/1 -> L1_WP/1
  Compare To Constant/1 -> Switch/2
  NearbyRefWP/2(d) -> Compare To Constant1/1  "distance"
  SearchL1RefWP/2(u) -> Compare To Constant/1  "l1_u"
  Compare To Constant1/1 -> Switch1/2
  P1/1 -> SearchL1RefWP/1(P1), OutRegionRegWP/1(P1)
  P2/1 -> SearchL1RefWP/2(P2), NearbyRefWP/1(P2), OutRegionRegWP/2(P2)
  P3/1 -> NearbyRefWP/2(P3), SearchL1RefWP/3(P3), OutRegionRegWP/3(P3)
  Switch/1 -> Switch1/3
  L1/1 -> SearchL1RefWP/4(L1), NearbyRefWP/3(L1)
  OutRegionRegWP/1(P) -> Switch/3  "out_WP"
  Switch1/1 -> Reshape/1
  SearchL1RefWP/1(P) -> Switch/1  "L1_Ref_P"
  NearbyRefWP/1(P) -> Switch1/1  "NearbyWP"

== system Formation_FMS2/FMS Commander/Commander/Form_Subsystem/FormMission/FormMission_SubSystem/Leader_Controller/Position Command/L1 Control/L1_Core ==
  p_vehicle : Inport
  L1_WP : Inport  Port=2
  L1 : Inport  Port=3
  Vg : Inport  Port=4
  L1_Lateral_Acceleration : Subsystem
  Subtract : Sum  Inputs=+-
  ay_cmd_mPs2 : Outport  VectorParamsAs1DForOutWhenUnconnected=off
  wires:
  L1_WP/1 -> Subtract/1
  p_vehicle/1 -> Subtract/2
  L1/1 -> L1_Lateral_Acceleration/1(L1)
  Vg/1 -> L1_Lateral_Acceleration/2(Vg)
  Subtract/1 -> L1_Lateral_Acceleration/3(l1_path)
  L1_Lateral_Acceleration/1(l1_a_cmd) -> ay_cmd_mPs2/1

== system Formation_FMS2/FMS Commander/Commander/Form_Subsystem/FormAssemble/Mission_SubSystem/Position Command/L1 Control/L1_Core/L1_Lateral_Acceleration/Included Angle ==
  vec1 : Inport
  vec2 : Inport  Port=2
  2D Cross Product : FC_Lib/Math/2D Cross Product
      settings: SourceProductName=Flight Control Toolbox
  Acos : Trigonometry  Operator=acos
  Constant4 : Constant  OutDataTypeStr=single
  Demux : Demux  Outputs=2
  Demux1 : Demux  Outputs=2
  Dot Product : DotProduct  OutDataTypeStr=Inherit: Inherit via internal rule
  Multiply : Product
  Mux : Mux  Inputs=2
  Mux1 : Mux  Inputs=2
  Sign1 : Signum
  Switch2 : Switch  Criteria=u2 ~= 0  SaturateOnIntegerOverflow=off  InputSameDT=off
  Vector Normalize : FC_Lib/Math/Vector Normalize
      settings: SourceProductName=Flight Control Toolbox
  Vector Normalize1 : FC_Lib/Math/Vector Normalize
      settings: SourceProductName=Flight Control Toolbox
  angle_rad : Outport  VectorParamsAs1DForOutWhenUnconnected=off
  wires:
  Switch2/1 -> Multiply/2
  Acos/1 -> Multiply/1
  Mux/1 -> Vector Normalize1/1
  vec2/1 -> Demux/1
  Constant4/1 -> Switch2/3
  Demux/1 -> Mux/2
  vec1/1 -> Demux1/1
  Multiply/1 -> angle_rad/1
  2D Cross Product/1 -> Sign1/1
  Vector Normalize/1 -> 2D Cross Product/2, Dot Product/1
  Demux/2 -> Mux/1
  Vector Normalize1/1 -> 2D Cross Product/1, Dot Product/2
  Sign1/1 -> Switch2/2, Switch2/1
  Demux1/2 -> Mux1/1
  Mux1/1 -> Vector Normalize/1
  Demux1/1 -> Mux1/2
  Dot Product/1 -> Acos/1

== system Formation_FMS2/FMS Commander/Commander/Form_Subsystem/FormMission/FormMission_SubSystem/Leader_Controller/Position Command/L1 Control/L1_Core/L1_Lateral_Acceleration ==
  L1 : Inport
  Vg : Inport  Port=2
  l1_path : Inport  Port=3
  Divide : Product  Inputs=*/
  Gain : Gain  Gain=2
  Included Angle : Subsystem
  Multiply1 : Product
  Saturation : Saturate  UpperLimit=pi/2  LowerLimit=-pi/2
  Sin : Trigonometry
  Square : Math  Operator=square  SignedPower=on
  Vector Modulus : FC_Lib/Math/Vector Modulus
      settings: SourceProductName=Flight Control Toolbox
  Vector Normalize : FC_Lib/Math/Vector Normalize
      settings: SourceProductName=Flight Control Toolbox
  Vector Normalize1 : FC_Lib/Math/Vector Normalize
      settings: SourceProductName=Flight Control Toolbox
  l1_a_cmd : Outport  VectorParamsAs1DForOutWhenUnconnected=off
  wires:
  Vector Normalize/1 -> Included Angle/1(vec1)
  Included Angle/1(angle_rad) -> Saturation/1  "L1_alpha"
  Multiply1/1 -> Divide/1
  Divide/1 -> l1_a_cmd/1  "l1_a_cmd"
  Vector Normalize1/1 -> Included Angle/2(vec2)
  Sin/1 -> Multiply1/1  "sin_alpha"
  l1_path/1 -> Vector Normalize1/1
  Saturation/1 -> Sin/1
  Vg/1 -> Vector Normalize/1, Vector Modulus/1
  Square/1 -> Gain/1
  Gain/1 -> Multiply1/2
  L1/1 -> Divide/2
  Vector Modulus/1 -> Square/1

== system Formation_FMS2/FMS Commander/Commander/Form_Subsystem/FormMission/FormMission_SubSystem/Leader_Controller/Position Command/L1 Control/L1_Core/L1_Lateral_Acceleration/Included Angle ==
  vec1 : Inport
  vec2 : Inport  Port=2
  2D Cross Product : FC_Lib/Math/2D Cross Product
      settings: SourceProductName=Flight Control Toolbox
  Acos : Trigonometry  Operator=acos
  Constant4 : Constant  OutDataTypeStr=single
  Demux : Demux  Outputs=2
  Demux1 : Demux  Outputs=2
  Dot Product : DotProduct  OutDataTypeStr=Inherit: Inherit via internal rule
  Multiply : Product
  Mux : Mux  Inputs=2
  Mux1 : Mux  Inputs=2
  Sign1 : Signum
  Switch2 : Switch  Criteria=u2 ~= 0  SaturateOnIntegerOverflow=off  InputSameDT=off
  Vector Normalize : FC_Lib/Math/Vector Normalize
      settings: SourceProductName=Flight Control Toolbox
  Vector Normalize1 : FC_Lib/Math/Vector Normalize
      settings: SourceProductName=Flight Control Toolbox
  angle_rad : Outport  VectorParamsAs1DForOutWhenUnconnected=off
  wires:
  Switch2/1 -> Multiply/2
  Acos/1 -> Multiply/1
  Mux/1 -> Vector Normalize1/1
  vec2/1 -> Demux/1
  Constant4/1 -> Switch2/3
  Demux/1 -> Mux/2
  vec1/1 -> Demux1/1
  Multiply/1 -> angle_rad/1
  2D Cross Product/1 -> Sign1/1
  Vector Normalize/1 -> 2D Cross Product/2, Dot Product/1
  Demux/2 -> Mux/1
  Vector Normalize1/1 -> 2D Cross Product/1, Dot Product/2
  Sign1/1 -> Switch2/2, Switch2/1
  Demux1/2 -> Mux1/1
  Mux1/1 -> Vector Normalize/1
  Demux1/1 -> Mux1/2
  Dot Product/1 -> Acos/1

== matlab function Formation_FMS2/FMS Commander/Commander/Default/Loiter_Control/L1 Reference WP/OutRegionRegWP ==
  data: P0 input; P output; P_Vehicle input; R input; L1 input; n input
% Find the reference waypoint when vehicle has no intersection with loicter circle.
%
% There are two region defined:
%   Region 1: The vehicle is outside of loiter circle
%   Region 2: The else situation
%
function P = OutRegionRefWP(P0, P_Vehicle, R, L1, n)

if sum((P_Vehicle-P0).^2) > R^2
    % outside of loiter circle, we just select P0 as P
    P = P0;
else
    % inside of loiter circle, we just let vehicle keep current direction
    P = P_Vehicle + n*L1;
end

== matlab function Formation_FMS2/FMS Commander/Commander/Default/Loiter_Control/L1 Reference WP/SearchL1RefWP ==
  data: P_0 input; P output; P_Vehicle input; R input; L1 input; n output
% Find reference waypoint (L1RefWP) on the loiter circle with origin at 
% P_0 and radius of R
%
% The idea is to calculate the intersection point of 2 circles (P_0:R and
% P_Vehicle:L1).
% Refer to: Knut Andreas Lie's Unstructured PEBI-grids Adapting to Geological Features in Subsurface Reservoirs
%
% Input:
%   P_0: loiter circle origin
%   P_Vehicle: vehicle position
%   R: loiter radius
%   L1: the L1 distance
% Output:
%   P: L1 reference waypoint
%   n: number of intersection points.
function [P, n] = SearchL1RefWP(P_0, P_Vehicle, R, L1)

C0 = P_Vehicle;
R0 = L1;
C1 = P_0;
R1 = R;
P = single([0;0]);

if C0(1)==C1(1) && C0(2)==C1(2) && R==L1
   % we have 2 same circle
   n = 0;
   return;
end

d = sqrt(sum((C1-C0).^2));
a = (d^2 + R0^2 - R1^2) / (2*d);

% n1 is perpendicular to n0
n0 = (C1-C0)/d;
n1 = [0 -1; 1 0] * n0;

if a^2 > R0^2
    % no intersection
    n = 0;
elseif a^2 == R0^2
    % only 1 intersection
    n = 1;
    P = C0 + a*n0;
else
    % 2 intersection
    n = 2;
    % we always choose the point with clockwise direction,
    % if wants anti-clockwise direction, choose h = -sqrt(R0^2 - a^2)
    h = sqrt(R0^2 - a^2);
    P = C0 + a*n0 + h*n1; 
end

== stateflow chart Formation_FMS2/FMS State Machine ==
  state Vehicle
    state Formation
      du:
      Cmd_In.form_valid = check_form_valid(Formation_Cross,INS_Out);
      state valid = check_form_valid(Formation_Cross,INS_Out) [function]
      state FormAssemble
        en:
        Cmd_In.sp_waypoint = [INS_Out.x_R; INS_Out.y_R; INS_Out.h_R];
        if uav_id == 1
        Other_Mission_Data = dubinsPath(Formation_Cross);
        end
        state Other_Mission_Data = dubinsPath(Formation_Cross) [function]
        state path_ratio = dubinsPathRatio(waypoints,pose,wp_index) [function] [commented out]
        state Output = testinf(Input) [function] [commented out]
        state Waypoint
          en:
          % set current waypoint to previous setpoint waypoint
          Cmd_In.cur_waypoint = Cmd_In.sp_waypoint;
          % Geodetic coordinates (latitude, longitude, and altitude), specified as an m-by-3 array in [degrees degrees meters]
          % Altitude add home(3) here because the altitude when takeoff could be non-zero
          % lla = [double(Mission_Data.x(wp_index))*1e-7, double(Mission_Data.y(wp_index))*1e-7, double(-(Mission_Data.z(wp_index) + home(3)))];
          % target waypoint
          Cmd_In.sp_waypoint = [Mission_Data.x(wp_index); Mission_Data.y(wp_index); Mission_Data.z(wp_index)];%LLA2FLAT(lla, llo, 0, 0);
          if Cmd_In.cur_waypoint(1:2)==Cmd_In.sp_waypoint(1:2)
          Cmd_In.sp_waypoint(1:2) = Cmd_In.sp_waypoint(1:2) + 0.01;  % Prevent P1P2 to nan.
          end
          waypoints = [Mission_Data.x(1:5) Mission_Data.y(1:5) deg2rad(Mission_Data.heading(1:5)) Mission_Data.ext1(1:5) Mission_Data.ext2(1:5)];
          %du:
          %ratio = dubinsPathRatio(waypoints, [INS_Out.x_R, INS_Out.y_R, INS_Out.psi], max(wp_index - 1, 1));
          %left_time = Mission_Data.ext2(5) * (1 - ratio) / norm([INS_Out.vn INS_Out.ve]);
        state NextWP
          en:
          state = VehicleState.FormAssemble;
        state WaitForUpdate
          en:
          Cmd_In.cur_waypoint = [INS_Out.x_R; INS_Out.y_R; INS_Out.h_R];
          state = VehicleState.FormHold;
        state Hold
          en:
          Cmd_In.cur_waypoint = Cmd_In.sp_waypoint;
          state = VehicleState.FormHold;
        (junction 206) -> (junction 197) : {wp_index = wp_index + 1;}
        (junction 197) -> Vehicle.Formation.FormAssemble.NextWP
        (junction 215) -> (junction 206)
        WaitForUpdate -> Vehicle.Formation.FormAssemble.NextWP [order 1] : [hasChanged(Mission_Data.timestamp) && Mission_Data.type == 1]{wp_index=1;}
        (default) -> WaitForUpdate
        Vehicle.Formation.FormAssemble.NextWP -> Vehicle.Formation.FormAssemble.Waypoint [order 1] : [wp_index <= Mission_Data.valid_items]
        Vehicle.Formation.FormAssemble.Waypoint -> (junction 215) : [norm([INS_Out.x_R;INS_Out.y_R]-Cmd_In.sp_waypoint(1:2)) <= accept_radius]
        Vehicle.Formation.FormAssemble.NextWP -> Hold [order 2]
      state FormMission
        en:
        % Reference location of latitude and longitude, specified as an m-by-2 array, in degrees
        % llo = [INS_Out.lat_0, INS_Out.lon_0] * (180/pi);
        % Upon enter Mission mode, set current position as setpoint waypoint
        Cmd_In.sp_waypoint = [INS_Out.x_R; INS_Out.y_R; INS_Out.h_R];
        state = VehicleState.FormMission;
        state NextWP
        state Waypoint
          en:
          % set current waypoint to previous setpoint waypoint
          Cmd_In.cur_waypoint = Cmd_In.sp_waypoint;
          % Geodetic coordinates (latitude, longitude, and altitude), specified as an m-by-3 array in [degrees degrees meters]
          % Altitude add home(3) here because the altitude when takeoff could be non-zero
          % lla = [double(Mission_Data.x(wp_index))*1e-7, double(Mission_Data.y(wp_index))*1e-7, double(-(Mission_Data.z(wp_index) + home(3)))];
          % target waypoint
          Cmd_In.sp_waypoint = [Mission_Data.x(wp_index); Mission_Data.y(wp_index); Mission_Data.z(wp_index)];%LLA2FLAT(lla, llo, 0, 0);
        state Follower
        (junction 83) -> (junction 82) : {wp_index = wp_index + 1;}
        (junction 82) -> Vehicle.Formation.FormMission.NextWP
        (junction 84) -> (junction 83)
        (default) -> Vehicle.Formation.FormMission.NextWP
        Vehicle.Formation.FormMission.NextWP -> Vehicle.Formation.FormMission.Waypoint [order 2] : [wp_index <= Mission_Data.valid_items]
        Vehicle.Formation.FormMission.Waypoint -> (junction 84) : [norm([INS_Out.x_R;INS_Out.y_R]-Cmd_In.sp_waypoint(1:2)) <= accept_radius]
        FormMission -> Vehicle.Formation.FormMission.NextWP : [hasChanged(Mission_Data.timestamp) && Mission_Data.type == 3]{wp_index=1;}
        Vehicle.Formation.FormMission.NextWP -> Follower [order 1] : [uav_id~=1]
      state FormDisband
        en:
        state=VehicleState.FormDisband;
      state InvalidMode
      WaitForUpdate -> (junction 295) [order 2] : [after(10, sec)]
      Hold -> FormMission : [Cmd_In.form_valid == sum(bitset(0, 1:3))]
      (junction 97) -> FormAssemble [order 1] : [mode==PilotMode.FormAssemble]
      (default) -> (junction 97)
      (junction 97) -> (junction 286) [order 2]
      (junction 286) -> FormMission [order 1] : [mode==PilotMode.FormMission && Cmd_In.form_valid == sum(bitset(0, 1:3))]
      (junction 286) -> (junction 288) [order 2]
      (junction 288) -> FormDisband [order 1] : [mode==PilotMode.FormDisband]
      (junction 288) -> InvalidMode [order 2]
      InvalidMode -> (junction 295)
    state Standby
      en:
      Cmd_In.cur_waypoint = [INS_Out.x_R; INS_Out.y_R; INS_Out.h_R];
      state = VehicleState.Hold;
    Vehicle -> (junction 62) : [hasChanged(mode) && mode ~= PilotMode.None]
    (default) -> (junction 62)
    (junction 62) -> Formation [order 1] : [any(mode==[PilotMode.FormAssemble,PilotMode.FormMission,PilotMode.FormDisband])]
    (junction 62) -> (junction 78) [order 2]
    (junction 78) -> Standby
    (junction 295) -> Standby
  data: Formation_Cross function_input Bus: Formation_Cross_Bus size=1; INS_Out function_input Bus: INS_Out_Bus size=1; valid function_output uint32 size=1; Formation_Cross function_input Bus: Formation_Cross_Bus size=1; Other_Mission_Data function_output Bus: Other_Mission_Data_Bus size=1; waypoints function_input double size=1; pose function_input double size=1; wp_index function_input double size=1; path_ratio function_output double size=1; Input function_input double size=1; Output function_output double size=1; INS_Out input Bus: INS_Out_Bus; Formation_Cross input; mode input Enum: PilotMode; Mission_Data input Bus: Mission_Data_Bus; state output Enum: VehicleState; Cmd_In output Bus: Commander_In_Bus size=1; wp_index output uint16; accept_radius input; Other_Mission_Data output Bus: Other_Mission_Data_Bus; waypoints local; uav_id parameter; form_radius parameter

== matlab function Formation_FMS2/FMS Commander/Commander/Form_Subsystem/FormMission/FormMission_SubSystem/Leader_Controller/Position Command/L1 Control/L1 Reference WP/NearbyRefWP ==
  data: P output; P2 input; d output; P3 input; L1 input
% Find the reference waypoint when vehicle (P3) is close to target (P2)
%
% If the vehicle is close to target (distance(P2,P3) < L1), select P2 as
% reference waypoint and return the distance, otherwise return -1.
function [P,d] = NearbyRefWP(P2, P3, L1)

P3P2 = P2 - P3;
dis = sqrt(sum(P3P2.^2));

if dis <= L1
    d = dis;
    % select P2 as reference WP
    P = P2;
else
    d = single(-1);
    % unset WP
    P = single([0; 0]);
end

== matlab function Formation_FMS2/FMS Commander/Commander/Hold/Loiter_Control/L1 Reference WP/OutRegionRegWP ==
  data: P0 input; P output; P_Vehicle input; R input; L1 input; n input
% Find the reference waypoint when vehicle has no intersection with loicter circle.
%
% There are two region defined:
%   Region 1: The vehicle is outside of loiter circle
%   Region 2: The else situation
%
function P = OutRegionRefWP(P0, P_Vehicle, R, L1, n)

if sum((P_Vehicle-P0).^2) > R^2
    % outside of loiter circle, we just select P0 as P
    P = P0;
else
    % inside of loiter circle, we just let vehicle keep current direction
    P = P_Vehicle + n*L1;
end
